simulink model "epidemia_3"  (R2019b)
settings: Solver=ode4  StartTime=0.0  StopTime=tk  FixedStep=1  RelTol=1e-3
values from neighbouring files (symbols this model uses):
  beta = 0.1    [glowny.m]
  D0 = 1    [glowny.m]    (also in glowny_wsp_var.m)
  eta = 1/70    (= 0.0142857142857)    [glowny.m]    (also in glowny_wsp_var.m)
  N = 38e6    (= 38000000)    [glowny.m]    (also in glowny_wsp_var.m)
  O0 = 0.2*N    (= 7600000)    [glowny.m]    (also in glowny_wsp_var.m)
  T = 14    [glowny.m]    (also in glowny_wsp_var.m)
  Z0 = D0/eta    (= 70)    [glowny.m]    (also in glowny_wsp_var.m)
settings Model: Creator=marci  LastModifiedBy=marci

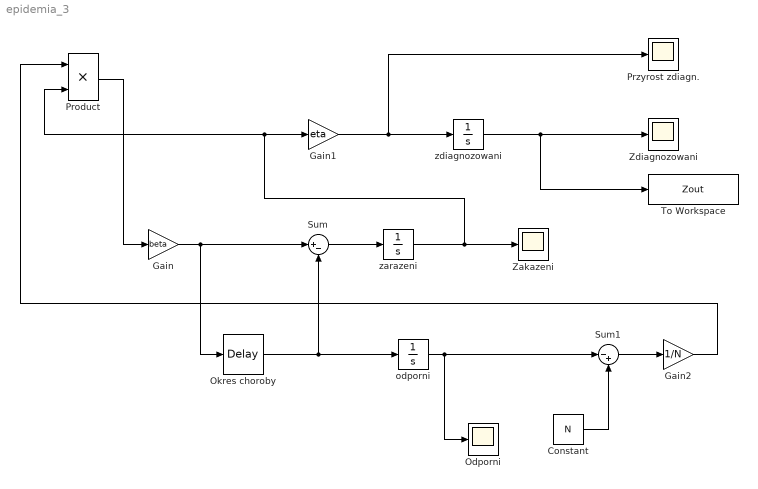
== system epidemia_3 ==
  Constant : Constant  Value=N
  Gain : Gain  Gain=beta
  Gain1 : Gain  Gain=eta
  Gain2 : Gain  Gain=1/N
  Odporni : Scope
  Okres choroby : TransportDelay  DelayTime=T
  Product : Product
  Przyrost zdiagn. : Scope
  Sum : Sum  Inputs=|+-
  Sum1 : Sum  Inputs=|-+
  To Workspace : ToWorkspace  VariableName=Zout  SaveFormat=Timeseries  SampleTime=-1
  Zakazeni : Scope
  Zdiagnozowani : Scope
  odporni : Integrator  InitialCondition=O0
  zarazeni : Integrator  InitialCondition=Z0  LimitOutput=on  UpperSaturationLimit=N  LowerSaturationLimit=0
  zdiagnozowani : Integrator  InitialCondition=D0
  wires:
  zarazeni/1 -> Zakazeni/1, Gain1/1, Product/2
  zdiagnozowani/1 -> To Workspace/1, Zdiagnozowani/1
  odporni/1 -> Odporni/1, Sum1/1
  Okres choroby/1 -> odporni/1, Sum/2
  Gain1/1 -> Przyrost zdiagn./1, zdiagnozowani/1
  Product/1 -> Gain/1
  Gain/1 -> Sum/1, Okres choroby/1
  Sum/1 -> zarazeni/1
  Sum1/1 -> Gain2/1
  Gain2/1 -> Product/1
  Constant/1 -> Sum1/2
